simulink model "Projeto_Final_versao_1_M21"  (R2021a)
settings: Solver=VariableStepAuto  StartTime=0  StopTime=144  FixedStep=0.1  RelTol=1e-3
model workspace (MAT data in the model file):
  N_P0 = 3
  variavelteste = 0
libraries: spsACVoltageSourceLib x1, spsCurrentMeasurementLib x1, spsSeriesRLCBranchLib x1, autolibsharedmappedengines x1, spspowerguiLib x1
(part 2 of 4)

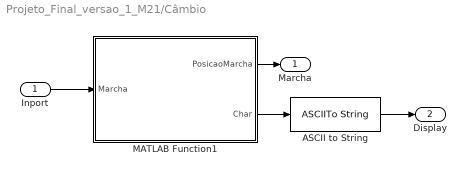
== system Projeto_Final_versao_1_M21/Câmbio ==
  Inport : Inport
  ASCII to String : ASCIIToString
  MATLAB Function1 : MATLAB Function  TreatAsAtomicUnit=on
  Marcha : Outport
  Display : Outport  Port=2
  wires:
  MATLAB Function1/1(PosicaoMarcha) -> Marcha/1
  MATLAB Function1/2(Char) -> ASCII to String/1
  ASCII to String/1 -> Display/1
  Inport/1 -> MATLAB Function1/1(Marcha)

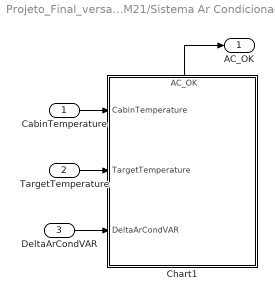
== system Projeto_Final_versao_1_M21/Sistema Ar Condicionado ==
  CabinTemperature : Inport
  TargetTemperature : Inport  Port=2
  DeltaArCondVAR : Inport  Port=3
  Chart1 : Stateflow chart  TreatAsAtomicUnit=on
      settings: PortSchema="{\"entries\":[{\"content\":{\"sides\":[{\"content\":{\"connectorIds\":[\"In1\",\"In2\",\"In3\"]},\"type\":\"ConnectorPlacement.EquallySpacedRectSide\",\"uuid\":\"3dcc586e-91d0-4cd1-aed7-6dda3adf5149\"},{\"content\":{\"connectorIds\":[],\"side\":\"RIGHT\"},\"type\":\"ConnectorPlacement.EquallySpacedRectSide\",\"uuid\":\"6a827bb4-538e-49ed-9fcc-bcf1675a0976\"},{\"content\":{\"connectorIds\":[\"Out1\"],\"side\":\"TOP\"},\"type\":\"ConnectorPlacement.EquallySpacedRectSide\",\"uuid\":\"8af03e4c-b384-4eb2-b8cc-d6be61dc8da4\"}]},\"type\":\"ConnectorPlacement.EquallySpacedConnector\",\"uuid\":\"bd7ebad6-2738-4989-9528-f935edcb496d\"}],\"packageUris\":[\"http://schema.mathworks.com/mf0/Connector/R2020b\"],\"version\":\"1.0\"}"
  AC_OK : Outport
  wires:
  Chart1/1(AC_OK) -> AC_OK/1
  CabinTemperature/1 -> Chart1/1(CabinTemperature)
  TargetTemperature/1 -> Chart1/2(TargetTemperature)
  DeltaArCondVAR/1 -> Chart1/3(DeltaArCondVAR)

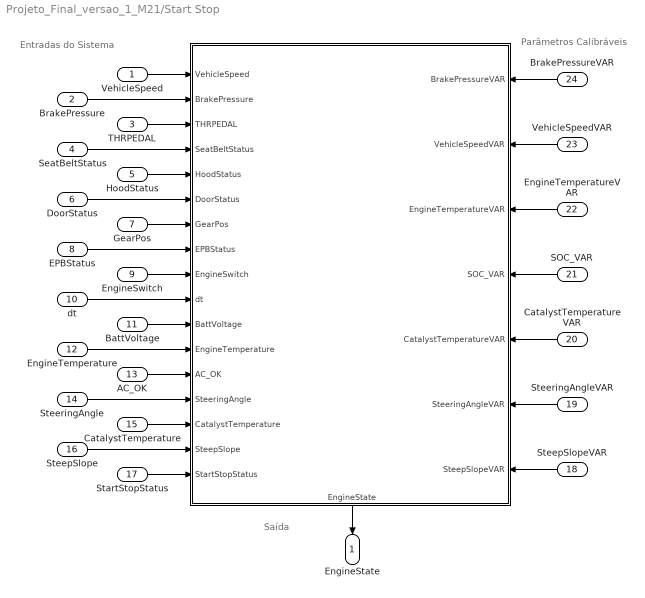
== system Projeto_Final_versao_1_M21/Start Stop ==
  note: Saída
  note: Entradas do Sistema
  note: Parâmetros Calibráveis
  VehicleSpeed : Inport
  BrakePressure : Inport  Port=2
  THRPEDAL : Inport  Port=3
  SeatBeltStatus : Inport  Port=4
  HoodStatus : Inport  Port=5
  DoorStatus : Inport  Port=6
  GearPos : Inport  Port=7
  EPBStatus : Inport  Port=8
  EngineSwitch : Inport  Port=9
  dt : Inport  Port=10
  BattVoltage : Inport  Port=11
  EngineTemperature : Inport  Port=12
  AC_OK : Inport  Port=13
  SteeringAngle : Inport  Port=14
  CatalystTemperature : Inport  Port=15
  SteepSlope : Inport  Port=16
  StartStopStatus : Inport  Port=17
  SteepSlopeVAR : Inport  Port=18
  SteeringAngleVAR : Inport  Port=19
  CatalystTemperatureVAR : Inport  Port=20
  SOC_VAR : Inport  Port=21
  EngineTemperatureVAR : Inport  Port=22
  VehicleSpeedVAR : Inport  Port=23
  BrakePressureVAR : Inport  Port=24
  " " : Stateflow chart  TreatAsAtomicUnit=on
      settings: PortSchema="{\"entries\":[{\"content\":{\"sides\":[{\"content\":{\"connectorIds\":[\"In8\",\"In9\",\"In10\",\"In11\",\"In12\",\"In13\",\"In14\",\"In15\",\"In16\",\"In17\",\"In18\",\"In19\",\"In20\",\"In21\",\"In22\",\"In23\",\"In24\"]},\"type\":\"ConnectorPlacement.EquallySpacedRectSide\",\"uuid\":\"823cfa7e-5a36-4c70-a231-0fae78490b25\"},{\"content\":{\"connectorIds\":[\"In1\",\"In2\",\"In3\",\"In4\",\"In5\",\"In6\",\"In7\"],\"side\":\"RIGHT\"},\"type\":\"ConnectorPlacement.EquallySpacedRectSide\",\"uuid\":\"b0c8ae88-7a9c-4152-8df4-361411c6999f\"},{\"content\":{\"connectorIds\":[],\"side\":\"TOP\"},\"type\":\"ConnectorPlacement.EquallySpacedRectSide\",\"uuid\":\"23b42440-538d-4cea-9d30-9fc9eba2f409\"},{\"content\":{\"connectorIds\":[\"Out1\"],\"side\":\"BOTTOM\"},\"type\":\"ConnectorPlacement.EquallySpacedRectSide\",\"uuid\":\"b132eeeb-9f39-4852-bf80-9b9b82940eba\"}]},\"type\":\"ConnectorPlacement.EquallySpacedConnector\",\"uuid\":\"9c597531-0edf-4da3-a7a2-f3937f962f4c\"}],\"packageUris\":[\"http://schema.mathworks.com/mf0/Connector/R2020b\"],\"version\":\"1.0\"}"
  EngineState : Outport
  wires:
  THRPEDAL/1 -> " "/10(THRPEDAL)
  EngineTemperature/1 -> " "/19(EngineTemperature)
  AC_OK/1 -> " "/20(AC_OK)
  BattVoltage/1 -> " "/18(BattVoltage)
  VehicleSpeed/1 -> " "/8(VehicleSpeed)
  GearPos/1 -> " "/14(GearPos)
  BrakePressure/1 -> " "/9(BrakePressure)
  dt/1 -> " "/17(dt)
  HoodStatus/1 -> " "/12(HoodStatus)
  DoorStatus/1 -> " "/13(DoorStatus)
  EngineSwitch/1 -> " "/16(EngineSwitch)
  EPBStatus/1 -> " "/15(EPBStatus)
  SeatBeltStatus/1 -> " "/11(SeatBeltStatus)
  SteeringAngle/1 -> " "/21(SteeringAngle)
  CatalystTemperature/1 -> " "/22(CatalystTemperature)
  SteepSlope/1 -> " "/23(SteepSlope)
  StartStopStatus/1 -> " "/24(StartStopStatus)
  " "/1(EngineState) -> EngineState/1
  SteepSlopeVAR/1 -> " "/7(SteepSlopeVAR)
  SteeringAngleVAR/1 -> " "/6(SteeringAngleVAR)
  CatalystTemperatureVAR/1 -> " "/5(CatalystTemperatureVAR)
  SOC_VAR/1 -> " "/4(SOC_VAR)
  EngineTemperatureVAR/1 -> " "/3(EngineTemperatureVAR)
  VehicleSpeedVAR/1 -> " "/2(VehicleSpeedVAR)
  BrakePressureVAR/1 -> " "/1(BrakePressureVAR)
